simulink model "PID_CL"  (R2024a)
settings: Solver=ode4  StartTime=0.0  StopTime=30  FixedStep=0.001  RelTol=1e-3
undefined symbols (not defined in the file or in its folder): Kd, Ki, Kp
libraries: simulink x2
settings Model: Creator=jhdac  LastModifiedBy=jhdac

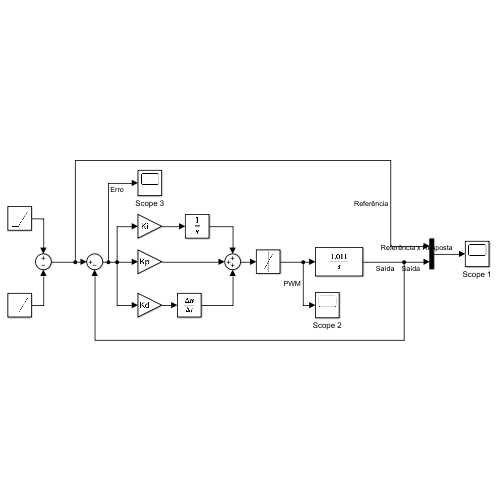
[thumbnail: Simulink's stored preview of the top-level diagram]
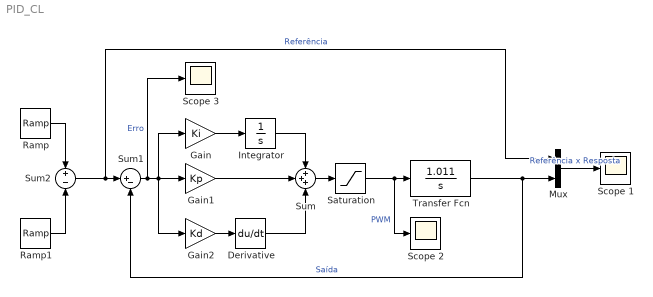
== system PID_CL ==
  Derivative : Derivative
  Gain : Gain  Gain=Ki
  Gain1 : Gain  Gain=Kp
  Gain2 : Gain  Gain=Kd
  Integrator : Integrator
  Mux : Mux  Inputs=2
  Ramp : simulink/Sources/Ramp  slope=250  start=0  InitialOutput=0
  Ramp1 : simulink/Sources/Ramp  slope=250  start=5  InitialOutput=0
  Saturation : Saturate  UpperLimit=255  LowerLimit=-255
  Scope 1 : Scope
  Scope 2 : Scope
  Scope 3 : Scope
  Sum : Sum  Inputs=+++
  Sum1 : Sum  Inputs=|+-
  Sum2 : Sum  Inputs=+-
  Transfer Fcn : TransferFcn  Numerator=[1.011]  Denominator=[1 0]
  wires:
  Sum1/1 -> Gain2/1, Gain1/1, Gain/1, Scope 3/1  "Erro"
  Gain1/1 -> Sum/2
  Integrator/1 -> Sum/1
  Sum/1 -> Saturation/1
  Gain/1 -> Integrator/1
  Mux/1 -> Scope 1/1  "Referência x Resposta"
  Ramp/1 -> Sum2/1
  Sum2/1 -> Mux/1, Sum1/1  "Referência"
  Transfer Fcn/1 -> Mux/2, Sum1/2  "Saída"
  Saturation/1 -> Scope 2/1, Transfer Fcn/1  "PWM"
  Ramp1/1 -> Sum2/2
  Gain2/1 -> Derivative/1
  Derivative/1 -> Sum/3
